simulink model "lab2ex5"  (R2020a)
settings: Solver=FixedStepDiscrete  StartTime=0.0  StopTime=65  RelTol=1e-3
settings Model: Creator=ace  LastModifiedBy=ace

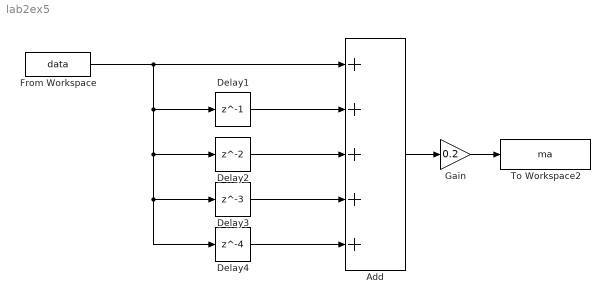
== system lab2ex5 ==
  Add : Sum  Inputs=+++++
  Delay1 : Delay  DelayLength=1  InitialCondition=0
  Delay2 : Delay  InitialCondition=0
  Delay3 : Delay  DelayLength=3  InitialCondition=0
  Delay4 : Delay  DelayLength=4  InitialCondition=0
  From Workspace : FromWorkspace  VariableName=data  SampleTime=1
  Gain : Gain  Gain=0.2
  To Workspace2 : ToWorkspace  VariableName=ma  SampleTime=1
  wires:
  From Workspace/1 -> Add/1, Delay4/1, Delay3/1, Delay2/1, Delay1/1
  Delay1/1 -> Add/2
  Delay2/1 -> Add/3
  Delay3/1 -> Add/4
  Delay4/1 -> Add/5
  Add/1 -> Gain/1
  Gain/1 -> To Workspace2/1
